simulink model "Sistema_mecanico_completo"  (R2023a)
settings: Solver=VariableStepAuto  StartTime=0.0  StopTime=10.0  RelTol=1e-3
undefined symbols (not defined in the file): b_eq, J_eq, k_l, L_d, L_q, lambda_m, Pp, r
settings Model: Creator=juanf  LastModifiedBy=juanf

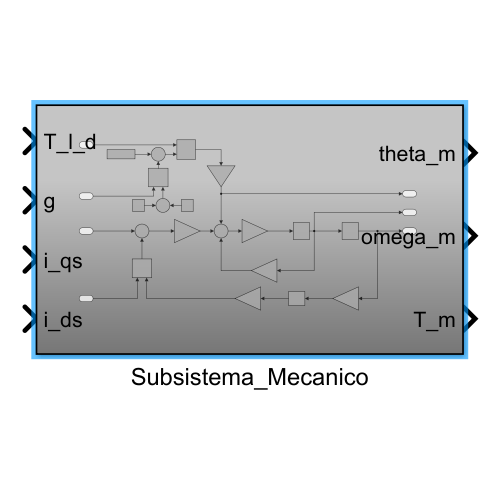
[thumbnail: Simulink's stored preview of the top-level diagram]
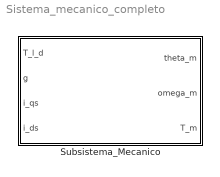
== system Sistema_mecanico_completo ==
  Subsistema_Mecanico : Subsystem

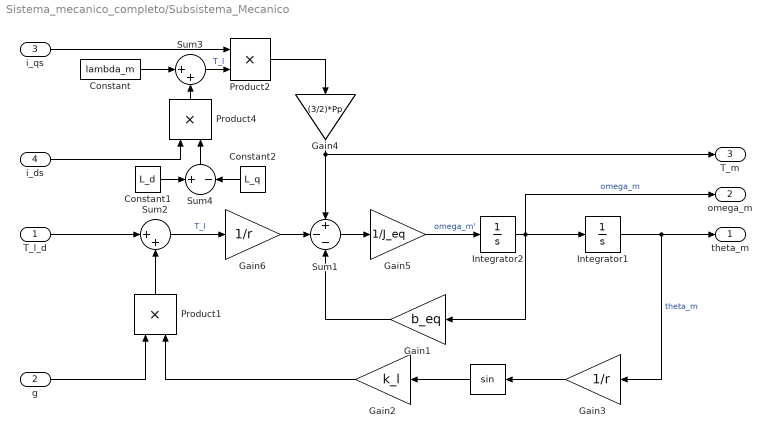
== system Sistema_mecanico_completo/Subsistema_Mecanico ==
  T_l_d : Inport
  g : Inport  Port=2
  i_qs : Inport  Port=3
  i_ds : Inport  Port=4
  " " : Trigonometry
  Constant : Constant  Value=lambda_m
  Constant1 : Constant  Value=L_d
  Constant2 : Constant  Value=L_q
  Gain1 : Gain  Gain=b_eq
  Gain2 : Gain  Gain=k_l
  Gain3 : Gain  Gain=1/r
  Gain4 : Gain  Gain=(3/2)*Pp
  Gain5 : Gain  Gain=1/J_eq
  Gain6 : Gain  Gain=1/r
  Integrator1 : Integrator
  Integrator2 : Integrator
  Product1 : Product
  Product2 : Product
  Product4 : Product
  Sum1 : Sum  Inputs=+--
  Sum2 : Sum  Inputs=|++
  Sum3 : Sum  Inputs=|++
  Sum4 : Sum  Inputs=+|-
  theta_m : Outport
  omega_m : Outport  Port=2
  T_m : Outport  Port=3
  wires:
  Product1/1 -> Sum2/2
  T_l_d/1 -> Sum2/1
  Integrator1/1 -> Gain3/1, theta_m/1  "theta_m"
  Gain3/1 -> " "/1
  " "/1 -> Gain2/1
  Gain1/1 -> Sum1/3
  Sum1/1 -> Gain5/1
  Sum2/1 -> Gain6/1  "T_l"
  Gain6/1 -> Sum1/2
  Integrator2/1 -> Gain1/1, omega_m/1, Integrator1/1  "omega_m"
  Gain5/1 -> Integrator2/1  "omega_m'"
  Gain2/1 -> Product1/2
  Gain4/1 -> T_m/1, Sum1/1
  g/1 -> Product1/1
  i_qs/1 -> Product2/1
  Product2/1 -> Gain4/1
  Constant/1 -> Sum3/1
  Product4/1 -> Sum3/2
  i_ds/1 -> Product4/1
  Sum4/1 -> Product4/2
  Constant2/1 -> Sum4/2
  Constant1/1 -> Sum4/1
  Sum3/1 -> Product2/2  "T_l"
